simulink model "model_2DOF"  (R2015a)
settings: Solver=ode45  StartTime=0.0  StopTime=10.0  RelTol=1e-3
undefined symbols (not defined in the file or in its folder): Ct, Dr, Jr, Mt
settings Model: Creator=shohei  LastModifiedBy=shohei

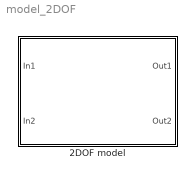
== system model_2DOF ==
  "2DOF model " : Subsystem

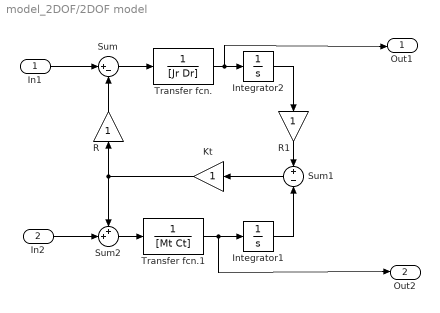
== system model_2DOF/2DOF model  ==
  In1 : Inport
  In2 : Inport  Port=2
  " Kt" : Gain
  Integrator1 : Integrator
  Integrator2 : Integrator
  R : Gain
  R1 : Gain
  Sum : Sum  Inputs=|+-
  Sum1 : Sum  Inputs=+|-
  Sum2 : Sum  Inputs=++|
  Transfer fcn. : TransferFcn  Denominator=[Jr Dr]
  Transfer fcn.1 : TransferFcn  Denominator=[Mt Ct]
  Out1 : Outport
  Out2 : Outport  Port=2
  wires:
  R/1 -> Sum/2
  Sum/1 -> Transfer fcn./1
  Transfer fcn./1 -> Out1/1, Integrator2/1
  R1/1 -> Sum1/1
  Integrator2/1 -> R1/1
  Sum1/1 -> " Kt"/1
  " Kt"/1 -> R/1, Sum2/1
  Sum2/1 -> Transfer fcn.1/1
  In2/1 -> Sum2/2
  In1/1 -> Sum/1
  Transfer fcn.1/1 -> Out2/1, Integrator1/1
  Integrator1/1 -> Sum1/2
